simulink model "tesv"  (R2012b)
settings: Solver=ode45  SolverMode=SingleTasking  StartTime=0.0  StopTime=10.0  RelTol=1e-3
libraries: xbsIndex_r4 x837
(part 1 of 6)
settings Model: Creator=tmadden  LastModifiedBy=tmadden
settings DataIOCC: SignalLoggingSaveFormat=ModelDataLogs
settings OptimizationCC: BlockReduction=off  BooleanDataType=off
settings DebuggingCC: SaveWithParameterizedLinksMsg=none  SignalResolutionControl=TryResolveAllWithWarning  SolverPrmCheckMsg=none  MultiTaskDSMMsg=warning  MultiTaskCondExecSysMsg=none  StrictBusMsg=None
settings HardwareCC: TargetUnknown=on
settings RTWCC: IncludeERTFirstTime=on

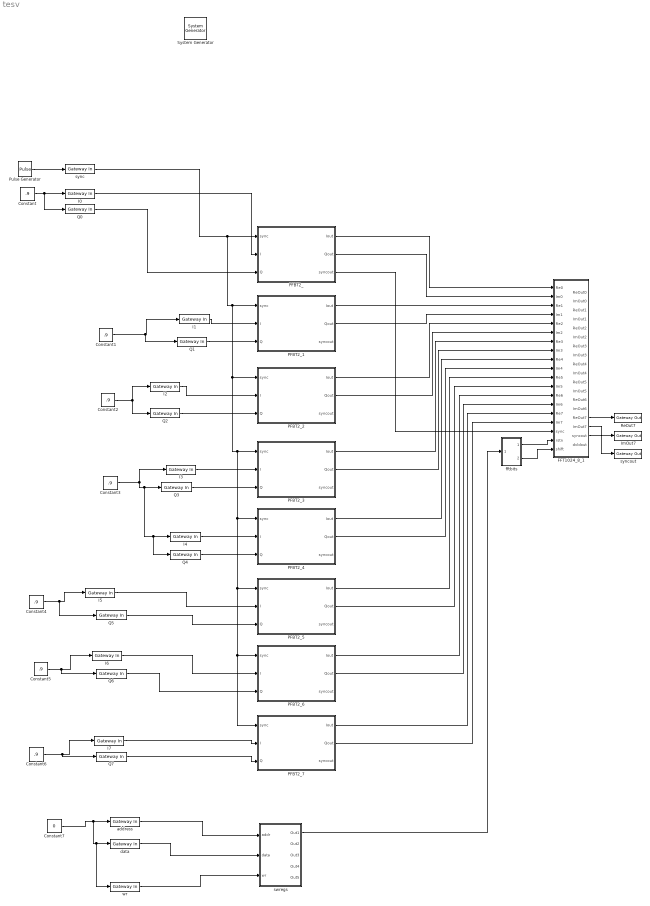
== system tesv ==
  " System Generator" : xbsIndex_r4/ System Generator  Tag=genX  xilinxfamily=zynq  part=xc7z100  speed=-2  package=ffv900  synthesis_tool=XST  clock_wrapper=Clock Enables  directory=./untitled/sysgen  proj_type=Project Navigator  Synth_file=XST Defaults  Impl_file=ISE Defaults  testbench=off  simulink_period=1  sysclk_period=10  dcm_input_clock_period=10  incr_netlist=off  trim_vbits=Everywhere in SubSystem  dbl_ovrd=According to Block Masks  core_generation=According to Block Masks  run_coregen=off  deprecated_control=off  eval_field=0  block_type=sysgen
  Constant{,1..6} (7 alike) : Constant  Value=.9
  Constant7 : Constant  Value=0
  FFT1024_8_1 : Subsystem
  I{0..7} (8 alike) : xbsIndex_r4/Gateway In  gui_display_data_type=Fixed-point  arith_type="Signed  (2's comp)"  n_bits=18  bin_pt=16  preci_type=Single  exp_width=8  frac_width=24  rows=1  columns=1  quantization="Round  (unbiased: +/- Inf)"  overflow=Saturate  period=1  UseAsADC=off  ADCChannel='1'  interface=None  automatic_assignment=on  address_offset=hex2dec('00')  intf_name=''  intf_description=''  timing_constraint=None  locs_specified=off  LOCs={}  io_standard={}  inherit_from_input=off  hdl_port=on  dbl_ovrd=off  block_type=gatewayin
  ImOut7 : xbsIndex_r4/Gateway Out  inherit_from_input=off  hdl_port=on  rows=1  columns=1  UseAsDAC=off  DACChannel='1'  interface=None  automatic_assignment=on  address_offset=hex2dec('00')  intf_name=''  intf_description=''  timing_constraint=None  locs_specified=off  LOCs={}  io_standard={}  block_type=gatewayout
  PFBT2_ : Subsystem
  PFBT2_1 : Subsystem
  PFBT2_2 : Subsystem
  PFBT2_3 : Subsystem
  PFBT2_4 : Subsystem
  PFBT2_5 : Subsystem
  PFBT2_6 : Subsystem
  PFBT2_7 : Subsystem
  Pulse Generator : DiscretePulseGenerator  Period=1024
  Q{0..7} (8 alike) : xbsIndex_r4/Gateway In  gui_display_data_type=Fixed-point  arith_type="Signed  (2's comp)"  n_bits=18  bin_pt=16  preci_type=Single  exp_width=8  frac_width=24  rows=1  columns=1  quantization="Round  (unbiased: +/- Inf)"  overflow=Saturate  period=1  UseAsADC=off  ADCChannel='1'  interface=None  automatic_assignment=on  address_offset=hex2dec('00')  intf_name=''  intf_description=''  timing_constraint=None  locs_specified=off  LOCs={}  io_standard={}  inherit_from_input=off  hdl_port=on  dbl_ovrd=off  block_type=gatewayin
  ReOut7 : xbsIndex_r4/Gateway Out  inherit_from_input=off  hdl_port=on  rows=1  columns=1  UseAsDAC=off  DACChannel='1'  interface=None  automatic_assignment=on  address_offset=hex2dec('00')  intf_name=''  intf_description=''  timing_constraint=None  locs_specified=off  LOCs={}  io_standard={}  block_type=gatewayout
  address : xbsIndex_r4/Gateway In  gui_display_data_type=Fixed-point  arith_type=Unsigned  n_bits=8  bin_pt=0  preci_type=Single  exp_width=8  frac_width=24  rows=1  columns=1  quantization="Round  (unbiased: +/- Inf)"  overflow=Saturate  period=1  UseAsADC=off  ADCChannel='1'  interface=None  automatic_assignment=on  address_offset=hex2dec('00')  intf_name=''  intf_description=''  timing_constraint=None  locs_specified=off  LOCs={}  io_standard={}  inherit_from_input=off  hdl_port=on  dbl_ovrd=off  block_type=gatewayin
  data : xbsIndex_r4/Gateway In  gui_display_data_type=Fixed-point  arith_type=Unsigned  n_bits=32  bin_pt=0  preci_type=Single  exp_width=8  frac_width=24  rows=1  columns=1  quantization="Round  (unbiased: +/- Inf)"  overflow=Saturate  period=1  UseAsADC=off  ADCChannel='1'  interface=None  automatic_assignment=on  address_offset=hex2dec('00')  intf_name=''  intf_description=''  timing_constraint=None  locs_specified=off  LOCs={}  io_standard={}  inherit_from_input=off  hdl_port=on  dbl_ovrd=off  block_type=gatewayin
  fftbits : Subsystem
  swregs : Subsystem
  sync : xbsIndex_r4/Gateway In  gui_display_data_type=Boolean  arith_type=Boolean  n_bits=16  bin_pt=14  preci_type=Single  exp_width=8  frac_width=24  rows=1  columns=1  quantization="Round  (unbiased: +/- Inf)"  overflow=Saturate  period=1  UseAsADC=off  ADCChannel='1'  interface=None  automatic_assignment=on  address_offset=hex2dec('00')  intf_name=''  intf_description=''  timing_constraint=None  locs_specified=off  LOCs={}  io_standard={}  inherit_from_input=off  hdl_port=on  dbl_ovrd=off  block_type=gatewayin
  syncout : xbsIndex_r4/Gateway Out  inherit_from_input=off  hdl_port=on  rows=1  columns=1  UseAsDAC=off  DACChannel='1'  interface=None  automatic_assignment=on  address_offset=hex2dec('00')  intf_name=''  intf_description=''  timing_constraint=None  locs_specified=off  LOCs={}  io_standard={}  block_type=gatewayout
  wr : xbsIndex_r4/Gateway In  gui_display_data_type=Boolean  arith_type=Boolean  n_bits=18  bin_pt=16  preci_type=Single  exp_width=8  frac_width=24  rows=1  columns=1  quantization="Round  (unbiased: +/- Inf)"  overflow=Saturate  period=1  UseAsADC=off  ADCChannel='1'  interface=None  automatic_assignment=on  address_offset=hex2dec('00')  intf_name=''  intf_description=''  timing_constraint=None  locs_specified=off  LOCs={}  io_standard={}  inherit_from_input=off  hdl_port=on  dbl_ovrd=off  block_type=gatewayin
  wires:
  Pulse Generator/1 -> sync/1
  Constant/1 -> Q0/1, I0/1
  sync/1 -> PFBT2_7/1(sync), PFBT2_6/1(sync), PFBT2_5/1(sync), PFBT2_4/1(sync), PFBT2_3/1(sync), PFBT2_2/1(sync), PFBT2_1/1(sync), PFBT2_/1(sync)
  I0/1 -> PFBT2_/2(I)
  Q0/1 -> PFBT2_/3(Q)
  I1/1 -> PFBT2_1/2(I)
  Q1/1 -> PFBT2_1/3(Q)
  I2/1 -> PFBT2_2/2(I)
  Q2/1 -> PFBT2_2/3(Q)
  I3/1 -> PFBT2_3/2(I)
  Q3/1 -> PFBT2_3/3(Q)
  I4/1 -> PFBT2_4/2(I)
  Q4/1 -> PFBT2_4/3(Q)
  I5/1 -> PFBT2_5/2(I)
  Q5/1 -> PFBT2_5/3(Q)
  I6/1 -> PFBT2_6/2(I)
  Q6/1 -> PFBT2_6/3(Q)
  I7/1 -> PFBT2_7/2(I)
  Q7/1 -> PFBT2_7/3(Q)
  Constant6/1 -> Q7/1, I7/1
  Constant5/1 -> Q6/1, I6/1
  Constant4/1 -> Q5/1, I5/1
  Constant3/1 -> Q4/1, I4/1, Q3/1, I3/1
  Constant1/1 -> Q1/1, I1/1
  Constant2/1 -> Q2/1, I2/1
  address/1 -> swregs/1(addr)
  data/1 -> swregs/2(data)
  wr/1 -> swregs/3(wr)
  PFBT2_/1(Iout) -> FFT1024_8_1/1(Re0)
  PFBT2_/2(Qout) -> FFT1024_8_1/2(Im0)
  PFBT2_1/1(Iout) -> FFT1024_8_1/3(Re1)
  PFBT2_1/2(Qout) -> FFT1024_8_1/4(Im1)
  PFBT2_2/1(Iout) -> FFT1024_8_1/5(Re2)
  PFBT2_2/2(Qout) -> FFT1024_8_1/6(Im2)
  PFBT2_3/1(Iout) -> FFT1024_8_1/7(Re3)
  PFBT2_3/2(Qout) -> FFT1024_8_1/8(Im3)
  PFBT2_4/1(Iout) -> FFT1024_8_1/9(Re4)
  PFBT2_4/2(Qout) -> FFT1024_8_1/10(Im4)
  PFBT2_5/1(Iout) -> FFT1024_8_1/11(Re5)
  PFBT2_5/2(Qout) -> FFT1024_8_1/12(Im5)
  PFBT2_6/1(Iout) -> FFT1024_8_1/13(Re6)
  PFBT2_6/2(Qout) -> FFT1024_8_1/14(Im6)
  PFBT2_7/1(Iout) -> FFT1024_8_1/15(Re7)
  PFBT2_7/2(Qout) -> FFT1024_8_1/16(Im7)
  PFBT2_/3(syncout) -> FFT1024_8_1/17(sync)
  fftbits/1(Out1) -> FFT1024_8_1/18(rstn)
  fftbits/2(Out2) -> FFT1024_8_1/19(shift)
  swregs/1(Out1) -> fftbits/1(In1)
  Constant7/1 -> wr/1, data/1, address/1
  FFT1024_8_1/15(ReOut7) -> ReOut7/1
  FFT1024_8_1/16(ImOut7) -> ImOut7/1
  FFT1024_8_1/17(syncout) -> syncout/1

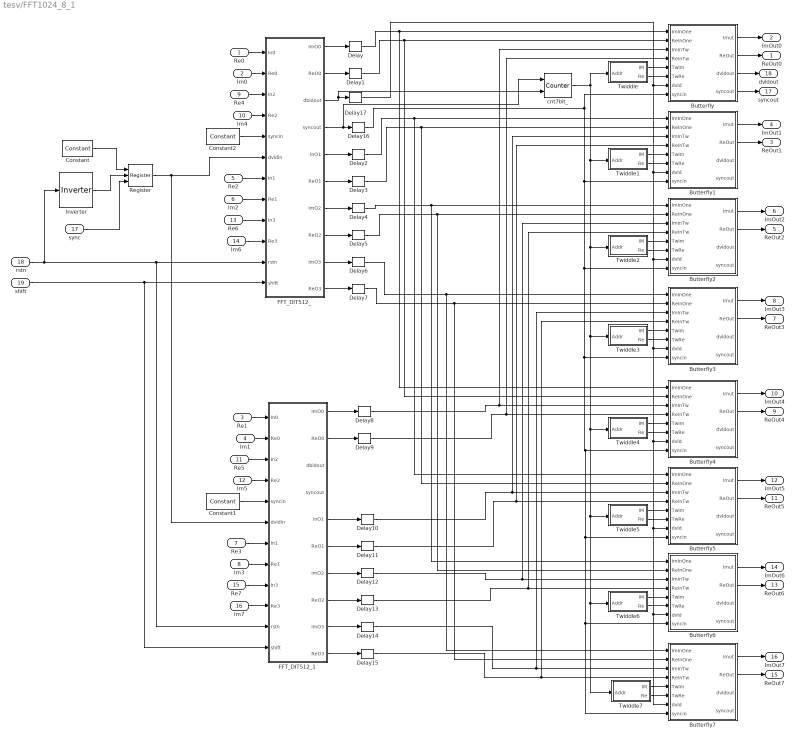
== system tesv/FFT1024_8_1 ==
  Re0 : Inport
  Im0 : Inport  Port=2
  Re1 : Inport  Port=3
  Im1 : Inport  Port=4
  Re2 : Inport  Port=5
  Im2 : Inport  Port=6
  Re3 : Inport  Port=7
  Im3 : Inport  Port=8
  Re4 : Inport  Port=9
  Im4 : Inport  Port=10
  Re5 : Inport  Port=11
  Im5 : Inport  Port=12
  Re6 : Inport  Port=13
  Im6 : Inport  Port=14
  Re7 : Inport  Port=15
  Im7 : Inport  Port=16
  sync : Inport  Port=17
  rstn : Inport  Port=18
  shift : Inport  Port=19
  Butterfly : Subsystem
  Butterfly1 : Subsystem
  Butterfly2 : Subsystem
  Butterfly3 : Subsystem
  Butterfly4 : Subsystem
  Butterfly5 : Subsystem
  Butterfly6 : Subsystem
  Butterfly7 : Subsystem
  Constant : xbsIndex_r4/Constant  const=1  gui_display_data_type=Boolean  arith_type=Boolean  n_bits=16  bin_pt=14  preci_type=Single  exp_width=8  frac_width=24  explicit_period=on  period=1  equ=P=C  opselect=C  inp2=PCIN>>17  opr=+  inp1=P  carry=CIN  dbl_ovrd=off  block_type=constant
  Constant1 : xbsIndex_r4/Constant  const=0  gui_display_data_type=Boolean  arith_type=Boolean  n_bits=16  bin_pt=14  preci_type=Single  exp_width=8  frac_width=24  explicit_period=on  period=1  equ=P=C  opselect=C  inp2=PCIN>>17  opr=+  inp1=P  carry=CIN  dbl_ovrd=off  block_type=constant
  Constant2 : xbsIndex_r4/Constant  const=0  gui_display_data_type=Boolean  arith_type=Boolean  n_bits=16  bin_pt=14  preci_type=Single  exp_width=8  frac_width=24  explicit_period=on  period=1  equ=P=C  opselect=C  inp2=PCIN>>17  opr=+  inp1=P  carry=CIN  dbl_ovrd=off  block_type=constant
  Delay{,1..17} (18 alike) : xbsIndex_r4/Delay  rst=off  infoeditControl=Selection of Reset will increase slice count due to use of real FFs and instead of SRLs  en=off  latency=1  reg_retiming=off  dbl_ovrd=off  block_type=delay
  FFT_DIT512_ : Subsystem
  FFT_DIT512_1 : Subsystem
  Inverter : xbsIndex_r4/Inverter  en=off  latency=0  dbl_ovrd=off  block_type=inv
  Register : xbsIndex_r4/Register  init=0  rst=on  en=on  dbl_ovrd=off  block_type=register
  Twiddle : Subsystem  mask{TFL=1024, NS=8, WS=0}
      mask prompts: TFL "TotFFTLen"; NS "NStreams (1...N)"; WS "WhichStream (0..N-1)"
  Twiddle1 : Subsystem  mask{TFL=1024, NS=8, WS=1}
      mask prompts: TFL "TotFFTLen"; NS "NStreams (1...N)"; WS "WhichStream (0..N-1)"
  Twiddle2 : Subsystem  mask{TFL=1024, NS=8, WS=2}
      mask prompts: TFL "TotFFTLen"; NS "NStreams (1...N)"; WS "WhichStream (0..N-1)"
  Twiddle3 : Subsystem  mask{TFL=1024, NS=8, WS=3}
      mask prompts: TFL "TotFFTLen"; NS "NStreams (1...N)"; WS "WhichStream (0..N-1)"
  Twiddle4 : Subsystem  mask{TFL=1024, NS=8, WS=4}
      mask prompts: TFL "TotFFTLen"; NS "NStreams (1...N)"; WS "WhichStream (0..N-1)"
  Twiddle5 : Subsystem  mask{TFL=1024, NS=8, WS=5}
      mask prompts: TFL "TotFFTLen"; NS "NStreams (1...N)"; WS "WhichStream (0..N-1)"
  Twiddle6 : Subsystem  mask{TFL=1024, NS=8, WS=6}
      mask prompts: TFL "TotFFTLen"; NS "NStreams (1...N)"; WS "WhichStream (0..N-1)"
  Twiddle7 : Subsystem  mask{TFL=1024, NS=8, WS=7}
      mask prompts: TFL "TotFFTLen"; NS "NStreams (1...N)"; WS "WhichStream (0..N-1)"
  cnt7bit_ : xbsIndex_r4/Counter  cnt_type=Free Running  cnt_to=Inf  operation=Up  start_count=0  cnt_by_val=1  arith_type=Unsigned  n_bits=log2(1024/8)  bin_pt=0  load_pin=off  rst=on  en=on  explicit_period=on  period=1  use_behavioral_HDL=off  implementation=Fabric  dbl_ovrd=off  block_type=counter
  ReOut0 : Outport
  ImOut0 : Outport  Port=2
  ReOut1 : Outport  Port=3
  ImOut1 : Outport  Port=4
  ReOut2 : Outport  Port=5
  ImOut2 : Outport  Port=6
  ReOut3 : Outport  Port=7
  ImOut3 : Outport  Port=8
  ReOut4 : Outport  Port=9
  ImOut4 : Outport  Port=10
  ReOut5 : Outport  Port=11
  ImOut5 : Outport  Port=12
  ReOut6 : Outport  Port=13
  ImOut6 : Outport  Port=14
  ReOut7 : Outport  Port=15
  ImOut7 : Outport  Port=16
  syncout : Outport  Port=17
  dvldout : Outport  Port=18
  wires:
  FFT_DIT512_/1(ImO0) -> Delay/1
  FFT_DIT512_/2(ReO0) -> Delay1/1
  Delay/1 -> Butterfly4/1(ImInOne), Butterfly/1(ImInOne)
  Delay1/1 -> Butterfly4/2(ReInOne), Butterfly/2(ReInOne)
  FFT_DIT512_/5(InO1) -> Delay2/1
  Delay2/1 -> Butterfly5/1(ImInOne), Butterfly1/1(ImInOne)
  Delay3/1 -> Butterfly5/2(ReInOne), Butterfly1/2(ReInOne)
  FFT_DIT512_/6(ReO1) -> Delay3/1
  Delay4/1 -> Butterfly6/1(ImInOne), Butterfly2/1(ImInOne)
  Delay5/1 -> Butterfly6/2(ReInOne), Butterfly2/2(ReInOne)
  FFT_DIT512_/7(ImO2) -> Delay4/1
  FFT_DIT512_/8(ReO2) -> Delay5/1
  FFT_DIT512_/9(ImO3) -> Delay6/1
  FFT_DIT512_/10(ReO3) -> Delay7/1
  Delay6/1 -> Butterfly7/1(ImInOne), Butterfly3/1(ImInOne)
  Delay7/1 -> Butterfly7/2(ReInOne), Butterfly3/2(ReInOne)
  FFT_DIT512_1/1(ImO0) -> Delay8/1
  FFT_DIT512_1/2(ReO0) -> Delay9/1
  FFT_DIT512_1/5(InO1) -> Delay10/1
  FFT_DIT512_1/6(ReO1) -> Delay11/1
  FFT_DIT512_1/7(ImO2) -> Delay12/1
  FFT_DIT512_1/8(ReO2) -> Delay13/1
  FFT_DIT512_1/9(ImO3) -> Delay14/1
  FFT_DIT512_1/10(ReO3) -> Delay15/1
  Delay8/1 -> Butterfly/3(ImInTw), Butterfly4/3(ImInTw)
  Delay9/1 -> Butterfly/4(ReInTw), Butterfly4/4(ReInTw)
  Delay10/1 -> Butterfly1/3(ImInTw), Butterfly5/3(ImInTw)
  Delay11/1 -> Butterfly1/4(ReInTw), Butterfly5/4(ReInTw)
  Delay12/1 -> Butterfly2/3(ImInTw), Butterfly6/3(ImInTw)
  Delay13/1 -> Butterfly2/4(ReInTw), Butterfly6/4(ReInTw)
  Delay14/1 -> Butterfly3/3(ImInTw), Butterfly7/3(ImInTw)
  Delay15/1 -> Butterfly3/4(ReInTw), Butterfly7/4(ReInTw)
  Twiddle7/1(IM) -> Butterfly7/5(TwIm)
  Twiddle7/2(Re) -> Butterfly7/6(TwRe)
  Twiddle6/1(IM) -> Butterfly6/5(TwIm)
  Twiddle6/2(Re) -> Butterfly6/6(TwRe)
  Twiddle5/1(IM) -> Butterfly5/5(TwIm)
  Twiddle5/2(Re) -> Butterfly5/6(TwRe)
  Twiddle4/1(IM) -> Butterfly4/5(TwIm)
  Twiddle4/2(Re) -> Butterfly4/6(TwRe)
  Twiddle/1(IM) -> Butterfly/5(TwIm)
  Twiddle/2(Re) -> Butterfly/6(TwRe)
  Twiddle1/1(IM) -> Butterfly1/5(TwIm)
  Twiddle1/2(Re) -> Butterfly1/6(TwRe)
  Twiddle2/1(IM) -> Butterfly2/5(TwIm)
  Twiddle2/2(Re) -> Butterfly2/6(TwRe)
  Twiddle3/1(IM) -> Butterfly3/5(TwIm)
  Twiddle3/2(Re) -> Butterfly3/6(TwRe)
  cnt7bit_/1 -> Twiddle/1(Addr), Twiddle7/1(Addr), Twiddle6/1(Addr), Twiddle5/1(Addr), Twiddle4/1(Addr), Twiddle3/1(Addr), Twiddle2/1(Addr), Twiddle1/1(Addr)
  Inverter/1 -> Register/2
  Constant/1 -> Register/1
  Constant2/1 -> FFT_DIT512_/5(syncin)
  Constant1/1 -> FFT_DIT512_1/5(syncin)
  Register/1 -> FFT_DIT512_1/6(dvldin), FFT_DIT512_/6(dvldin)
  FFT_DIT512_/4(syncout) -> cnt7bit_/1, Delay16/1
  Delay16/1 -> Butterfly7/8(syncin), Butterfly6/8(syncin), Butterfly5/8(syncin), Butterfly4/8(syncin), Butterfly3/8(syncin), Butterfly2/8(syncin), Butterfly1/8(syncin), Butterfly/8(syncin)
  FFT_DIT512_/3(dbldout) -> Delay17/1, cnt7bit_/2
  Delay17/1 -> Butterfly7/7(dvld), Butterfly6/7(dvld), Butterfly5/7(dvld), Butterfly4/7(dvld), Butterfly3/7(dvld), Butterfly2/7(dvld), Butterfly1/7(dvld), Butterfly/7(dvld)
  Im7/1 -> FFT_DIT512_1/10(Re3)
  Re7/1 -> FFT_DIT512_1/9(In3)
  Re3/1 -> FFT_DIT512_1/7(In1)
  Im3/1 -> FFT_DIT512_1/8(Re1)
  Im5/1 -> FFT_DIT512_1/4(Re2)
  Re5/1 -> FFT_DIT512_1/3(In2)
  Im1/1 -> FFT_DIT512_1/2(Re0)
  Re1/1 -> FFT_DIT512_1/1(In0)
  Im6/1 -> FFT_DIT512_/10(Re3)
  Re6/1 -> FFT_DIT512_/9(In3)
  Im2/1 -> FFT_DIT512_/8(Re1)
  Re2/1 -> FFT_DIT512_/7(In1)
  Re0/1 -> FFT_DIT512_/1(In0)
  Im0/1 -> FFT_DIT512_/2(Re0)
  Re4/1 -> FFT_DIT512_/3(In2)
  Im4/1 -> FFT_DIT512_/4(Re2)
  sync/1 -> Register/3
  rstn/1 -> Inverter/1, FFT_DIT512_1/11(rstn), FFT_DIT512_/11(rstn)
  shift/1 -> FFT_DIT512_1/12(shift), FFT_DIT512_/12(shift)
  Butterfly/2(ReOut) -> ReOut0/1
  Butterfly/1(Imut) -> ImOut0/1
  Butterfly1/1(Imut) -> ImOut1/1
  Butterfly1/2(ReOut) -> ReOut1/1
  Butterfly2/1(Imut) -> ImOut2/1
  Butterfly2/2(ReOut) -> ReOut2/1
  Butterfly3/1(Imut) -> ImOut3/1
  Butterfly3/2(ReOut) -> ReOut3/1
  Butterfly4/1(Imut) -> ImOut4/1
  Butterfly4/2(ReOut) -> ReOut4/1
  Butterfly5/1(Imut) -> ImOut5/1
  Butterfly5/2(ReOut) -> ReOut5/1
  Butterfly6/1(Imut) -> ImOut6/1
  Butterfly6/2(ReOut) -> ReOut6/1
  Butterfly7/1(Imut) -> ImOut7/1
  Butterfly7/2(ReOut) -> ReOut7/1
  Butterfly/3(dvldout) -> dvldout/1
  Butterfly/4(syncout) -> syncout/1

== system tesv/PFBT2_ ==
  sync : Inport
  I : Inport  Port=2
  Q : Inport  Port=3
  AddSub : xbsIndex_r4/AddSub  mode=Addition  use_carryin=off  use_carryout=off  en=off  latency=1  precision=Full  arith_type=Unsigned  n_bits=16  bin_pt=14  quantization=Truncate  overflow=Wrap  use_behavioral_HDL=off  hw_selection=Fabric  pipelined=off  dbl_ovrd=off  block_type=addsub
  AddSub1 : xbsIndex_r4/AddSub  mode=Addition  use_carryin=off  use_carryout=off  en=off  latency=1  precision=Full  arith_type=Unsigned  n_bits=16  bin_pt=14  quantization=Truncate  overflow=Wrap  use_behavioral_HDL=off  hw_selection=Fabric  pipelined=off  dbl_ovrd=off  block_type=addsub
  CoefAddr_ : Subsystem  mask{FL=1024, NS=8}
      mask prompts: FL "FilterLen (FFT Len)"; NS "NumStreams"
  Delay_ : Subsystem  mask{FL=1024, NS=8}
      mask prompts: FL "FiltLen (FFT Len)"; NS "NumStreams"
  Delay_1 : Subsystem  mask{FL=1024, NS=8}
      mask prompts: FL "FiltLen (FFT Len)"; NS "NumStreams"
  TapIQ_1 : Subsystem  mask{FL=1024, WS=0, NS=8, WT=1, NT=2}
      mask prompts: FL "FilterLen"; WS "WhichStream(0..3)"; NS "NStreams"; WT "WhichTap (0..3)"; NT "NumTaps"
  TapIQ_2 : Subsystem  mask{FL=1024, WS=0, NS=8, WT=0, NT=2}
      mask prompts: FL "FilterLen"; WS "WhichStream(0..3)"; NS "NStreams"; WT "WhichTap (0..3)"; NT "NumTaps"
  Iout : Outport
  Qout : Outport  Port=2
  syncout : Outport  Port=3
  wires:
  TapIQ_1/4(syncout) -> syncout/1
  Delay_/1(Iout) -> TapIQ_1/1(Iin)
  Delay_/2(Qout) -> TapIQ_1/2(Qin)
  TapIQ_2/1(Iout) -> Delay_1/1(Iin)
  TapIQ_1/1(Iout) -> AddSub/2
  Delay_1/1(Iout) -> AddSub/1
  Delay_1/2(Qout) -> AddSub1/1
  TapIQ_1/2(Qout) -> AddSub1/2
  Delay_/3(addrout) -> TapIQ_1/3(coefaddr)
  CoefAddr_/1(Addr) -> Delay_/3(addrin), TapIQ_2/3(coefaddr)
  Q/1 -> CoefAddr_/3(Qin)
  I/1 -> CoefAddr_/2(Iin)
  sync/1 -> CoefAddr_/1(sync)
  CoefAddr_/2(Iout) -> TapIQ_2/1(Iin), Delay_/1(Iin)
  CoefAddr_/3(Qout) -> Delay_/2(Qin), TapIQ_2/2(Qin)
  TapIQ_2/4(syncout) -> Delay_1/4(sync)
  CoefAddr_/4(syncout) -> TapIQ_2/4(sync), Delay_/4(sync)
  Delay_/4(syncout) -> TapIQ_1/4(sync)
  AddSub/1 -> Iout/1
  AddSub1/1 -> Qout/1
  TapIQ_2/2(Qout) -> Delay_1/2(Qin)
  TapIQ_2/3(coefaddrout) -> Delay_1/3(addrin)

== system tesv/PFBT2_1 ==
  sync : Inport
  I : Inport  Port=2
  Q : Inport  Port=3
  AddSub : xbsIndex_r4/AddSub  mode=Addition  use_carryin=off  use_carryout=off  en=off  latency=1  precision=Full  arith_type=Unsigned  n_bits=16  bin_pt=14  quantization=Truncate  overflow=Wrap  use_behavioral_HDL=off  hw_selection=Fabric  pipelined=off  dbl_ovrd=off  block_type=addsub
  AddSub1 : xbsIndex_r4/AddSub  mode=Addition  use_carryin=off  use_carryout=off  en=off  latency=1  precision=Full  arith_type=Unsigned  n_bits=16  bin_pt=14  quantization=Truncate  overflow=Wrap  use_behavioral_HDL=off  hw_selection=Fabric  pipelined=off  dbl_ovrd=off  block_type=addsub
  CoefAddr_ : Subsystem  mask{FL=1024, NS=8}
      mask prompts: FL "FilterLen (FFT Len)"; NS "NumStreams"
  Delay_ : Subsystem  mask{FL=1024, NS=8}
      mask prompts: FL "FiltLen (FFT Len)"; NS "NumStreams"
  Delay_1 : Subsystem  mask{FL=1024, NS=8}
      mask prompts: FL "FiltLen (FFT Len)"; NS "NumStreams"
  TapIQ_1 : Subsystem  mask{FL=1024, WS=1, NS=8, WT=1, NT=2}
      mask prompts: FL "FilterLen"; WS "WhichStream(0..3)"; NS "NStreams"; WT "WhichTap (0..3)"; NT "NumTaps"
  TapIQ_2 : Subsystem  mask{FL=1024, WS=1, NS=8, WT=0, NT=2}
      mask prompts: FL "FilterLen"; WS "WhichStream(0..3)"; NS "NStreams"; WT "WhichTap (0..3)"; NT "NumTaps"
  Iout : Outport
  Qout : Outport  Port=2
  syncout : Outport  Port=3
  wires:
  TapIQ_1/4(syncout) -> syncout/1
  Delay_/1(Iout) -> TapIQ_1/1(Iin)
  Delay_/2(Qout) -> TapIQ_1/2(Qin)
  TapIQ_2/1(Iout) -> Delay_1/1(Iin)
  TapIQ_1/1(Iout) -> AddSub/2
  Delay_1/1(Iout) -> AddSub/1
  Delay_1/2(Qout) -> AddSub1/1
  TapIQ_1/2(Qout) -> AddSub1/2
  Delay_/3(addrout) -> TapIQ_1/3(coefaddr)
  CoefAddr_/1(Addr) -> Delay_/3(addrin), TapIQ_2/3(coefaddr)
  Q/1 -> CoefAddr_/3(Qin)
  I/1 -> CoefAddr_/2(Iin)
  sync/1 -> CoefAddr_/1(sync)
  CoefAddr_/2(Iout) -> TapIQ_2/1(Iin), Delay_/1(Iin)
  CoefAddr_/3(Qout) -> Delay_/2(Qin), TapIQ_2/2(Qin)
  TapIQ_2/4(syncout) -> Delay_1/4(sync)
  CoefAddr_/4(syncout) -> TapIQ_2/4(sync), Delay_/4(sync)
  Delay_/4(syncout) -> TapIQ_1/4(sync)
  AddSub/1 -> Iout/1
  AddSub1/1 -> Qout/1
  TapIQ_2/2(Qout) -> Delay_1/2(Qin)
  TapIQ_2/3(coefaddrout) -> Delay_1/3(addrin)

== system tesv/PFBT2_2 ==
  sync : Inport
  I : Inport  Port=2
  Q : Inport  Port=3
  AddSub : xbsIndex_r4/AddSub  mode=Addition  use_carryin=off  use_carryout=off  en=off  latency=1  precision=Full  arith_type=Unsigned  n_bits=16  bin_pt=14  quantization=Truncate  overflow=Wrap  use_behavioral_HDL=off  hw_selection=Fabric  pipelined=off  dbl_ovrd=off  block_type=addsub
  AddSub1 : xbsIndex_r4/AddSub  mode=Addition  use_carryin=off  use_carryout=off  en=off  latency=1  precision=Full  arith_type=Unsigned  n_bits=16  bin_pt=14  quantization=Truncate  overflow=Wrap  use_behavioral_HDL=off  hw_selection=Fabric  pipelined=off  dbl_ovrd=off  block_type=addsub
  CoefAddr_ : Subsystem  mask{FL=1024, NS=8}
      mask prompts: FL "FilterLen (FFT Len)"; NS "NumStreams"
  Delay_ : Subsystem  mask{FL=512, NS=2}
      mask prompts: FL "FiltLen (FFT Len)"; NS "NumStreams"
  Delay_1 : Subsystem  mask{FL=1024, NS=8}
      mask prompts: FL "FiltLen (FFT Len)"; NS "NumStreams"
  TapIQ_1 : Subsystem  mask{FL=1024, WS=2, NS=8, WT=1, NT=2}
      mask prompts: FL "FilterLen"; WS "WhichStream(0..3)"; NS "NStreams"; WT "WhichTap (0..3)"; NT "NumTaps"
  TapIQ_2 : Subsystem  mask{FL=1024, WS=2, NS=8, WT=0, NT=2}
      mask prompts: FL "FilterLen"; WS "WhichStream(0..3)"; NS "NStreams"; WT "WhichTap (0..3)"; NT "NumTaps"
  Iout : Outport
  Qout : Outport  Port=2
  syncout : Outport  Port=3
  wires:
  TapIQ_1/4(syncout) -> syncout/1
  Delay_/1(Iout) -> TapIQ_1/1(Iin)
  Delay_/2(Qout) -> TapIQ_1/2(Qin)
  TapIQ_2/1(Iout) -> Delay_1/1(Iin)
  TapIQ_1/1(Iout) -> AddSub/2
  Delay_1/1(Iout) -> AddSub/1
  Delay_1/2(Qout) -> AddSub1/1
  TapIQ_1/2(Qout) -> AddSub1/2
  Delay_/3(addrout) -> TapIQ_1/3(coefaddr)
  CoefAddr_/1(Addr) -> Delay_/3(addrin), TapIQ_2/3(coefaddr)
  Q/1 -> CoefAddr_/3(Qin)
  I/1 -> CoefAddr_/2(Iin)
  sync/1 -> CoefAddr_/1(sync)
  CoefAddr_/2(Iout) -> TapIQ_2/1(Iin), Delay_/1(Iin)
  CoefAddr_/3(Qout) -> Delay_/2(Qin), TapIQ_2/2(Qin)
  TapIQ_2/4(syncout) -> Delay_1/4(sync)
  CoefAddr_/4(syncout) -> TapIQ_2/4(sync), Delay_/4(sync)
  Delay_/4(syncout) -> TapIQ_1/4(sync)
  AddSub/1 -> Iout/1
  AddSub1/1 -> Qout/1
  TapIQ_2/2(Qout) -> Delay_1/2(Qin)
  TapIQ_2/3(coefaddrout) -> Delay_1/3(addrin)

== system tesv/PFBT2_3 ==
  sync : Inport
  I : Inport  Port=2
  Q : Inport  Port=3
  AddSub : xbsIndex_r4/AddSub  mode=Addition  use_carryin=off  use_carryout=off  en=off  latency=1  precision=Full  arith_type=Unsigned  n_bits=16  bin_pt=14  quantization=Truncate  overflow=Wrap  use_behavioral_HDL=off  hw_selection=Fabric  pipelined=off  dbl_ovrd=off  block_type=addsub
  AddSub1 : xbsIndex_r4/AddSub  mode=Addition  use_carryin=off  use_carryout=off  en=off  latency=1  precision=Full  arith_type=Unsigned  n_bits=16  bin_pt=14  quantization=Truncate  overflow=Wrap  use_behavioral_HDL=off  hw_selection=Fabric  pipelined=off  dbl_ovrd=off  block_type=addsub
  CoefAddr_ : Subsystem  mask{FL=1024, NS=8}
      mask prompts: FL "FilterLen (FFT Len)"; NS "NumStreams"
  Delay_ : Subsystem  mask{FL=1024, NS=8}
      mask prompts: FL "FiltLen (FFT Len)"; NS "NumStreams"
  Delay_1 : Subsystem  mask{FL=1024, NS=8}
      mask prompts: FL "FiltLen (FFT Len)"; NS "NumStreams"
  TapIQ_1 : Subsystem  mask{FL=1024, WS=3, NS=8, WT=1, NT=2}
      mask prompts: FL "FilterLen"; WS "WhichStream(0..3)"; NS "NStreams"; WT "WhichTap (0..3)"; NT "NumTaps"
  TapIQ_2 : Subsystem  mask{FL=1024, WS=3, NS=8, WT=0, NT=2}
      mask prompts: FL "FilterLen"; WS "WhichStream(0..3)"; NS "NStreams"; WT "WhichTap (0..3)"; NT "NumTaps"
  Iout : Outport
  Qout : Outport  Port=2
  syncout : Outport  Port=3
  wires:
  TapIQ_1/4(syncout) -> syncout/1
  Delay_/1(Iout) -> TapIQ_1/1(Iin)
  Delay_/2(Qout) -> TapIQ_1/2(Qin)
  TapIQ_2/1(Iout) -> Delay_1/1(Iin)
  TapIQ_1/1(Iout) -> AddSub/2
  Delay_1/1(Iout) -> AddSub/1
  Delay_1/2(Qout) -> AddSub1/1
  TapIQ_1/2(Qout) -> AddSub1/2
  Delay_/3(addrout) -> TapIQ_1/3(coefaddr)
  CoefAddr_/1(Addr) -> Delay_/3(addrin), TapIQ_2/3(coefaddr)
  Q/1 -> CoefAddr_/3(Qin)
  I/1 -> CoefAddr_/2(Iin)
  sync/1 -> CoefAddr_/1(sync)
  CoefAddr_/2(Iout) -> TapIQ_2/1(Iin), Delay_/1(Iin)
  CoefAddr_/3(Qout) -> Delay_/2(Qin), TapIQ_2/2(Qin)
  TapIQ_2/4(syncout) -> Delay_1/4(sync)
  CoefAddr_/4(syncout) -> TapIQ_2/4(sync), Delay_/4(sync)
  Delay_/4(syncout) -> TapIQ_1/4(sync)
  AddSub/1 -> Iout/1
  AddSub1/1 -> Qout/1
  TapIQ_2/2(Qout) -> Delay_1/2(Qin)
  TapIQ_2/3(coefaddrout) -> Delay_1/3(addrin)

== system tesv/PFBT2_4 ==
  sync : Inport
  I : Inport  Port=2
  Q : Inport  Port=3
  AddSub : xbsIndex_r4/AddSub  mode=Addition  use_carryin=off  use_carryout=off  en=off  latency=1  precision=Full  arith_type=Unsigned  n_bits=16  bin_pt=14  quantization=Truncate  overflow=Wrap  use_behavioral_HDL=off  hw_selection=Fabric  pipelined=off  dbl_ovrd=off  block_type=addsub
  AddSub1 : xbsIndex_r4/AddSub  mode=Addition  use_carryin=off  use_carryout=off  en=off  latency=1  precision=Full  arith_type=Unsigned  n_bits=16  bin_pt=14  quantization=Truncate  overflow=Wrap  use_behavioral_HDL=off  hw_selection=Fabric  pipelined=off  dbl_ovrd=off  block_type=addsub
  CoefAddr_ : Subsystem  mask{FL=1024, NS=8}
      mask prompts: FL "FilterLen (FFT Len)"; NS "NumStreams"
  Delay_ : Subsystem  mask{FL=1024, NS=8}
      mask prompts: FL "FiltLen (FFT Len)"; NS "NumStreams"
  Delay_1 : Subsystem  mask{FL=1024, NS=8}
      mask prompts: FL "FiltLen (FFT Len)"; NS "NumStreams"
  TapIQ_1 : Subsystem  mask{FL=1024, WS=4, NS=8, WT=1, NT=2}
      mask prompts: FL "FilterLen"; WS "WhichStream(0..3)"; NS "NStreams"; WT "WhichTap (0..3)"; NT "NumTaps"
  TapIQ_2 : Subsystem  mask{FL=1024, WS=4, NS=8, WT=0, NT=2}
      mask prompts: FL "FilterLen"; WS "WhichStream(0..3)"; NS "NStreams"; WT "WhichTap (0..3)"; NT "NumTaps"
  Iout : Outport
  Qout : Outport  Port=2
  syncout : Outport  Port=3
  wires:
  TapIQ_1/4(syncout) -> syncout/1
  Delay_/1(Iout) -> TapIQ_1/1(Iin)
  Delay_/2(Qout) -> TapIQ_1/2(Qin)
  TapIQ_2/1(Iout) -> Delay_1/1(Iin)
  TapIQ_1/1(Iout) -> AddSub/2
  Delay_1/1(Iout) -> AddSub/1
  Delay_1/2(Qout) -> AddSub1/1
  TapIQ_1/2(Qout) -> AddSub1/2
  Delay_/3(addrout) -> TapIQ_1/3(coefaddr)
  CoefAddr_/1(Addr) -> Delay_/3(addrin), TapIQ_2/3(coefaddr)
  Q/1 -> CoefAddr_/3(Qin)
  I/1 -> CoefAddr_/2(Iin)
  sync/1 -> CoefAddr_/1(sync)
  CoefAddr_/2(Iout) -> TapIQ_2/1(Iin), Delay_/1(Iin)
  CoefAddr_/3(Qout) -> Delay_/2(Qin), TapIQ_2/2(Qin)
  TapIQ_2/4(syncout) -> Delay_1/4(sync)
  CoefAddr_/4(syncout) -> TapIQ_2/4(sync), Delay_/4(sync)
  Delay_/4(syncout) -> TapIQ_1/4(sync)
  AddSub/1 -> Iout/1
  AddSub1/1 -> Qout/1
  TapIQ_2/2(Qout) -> Delay_1/2(Qin)
  TapIQ_2/3(coefaddrout) -> Delay_1/3(addrin)

== system tesv/PFBT2_5 ==
  sync : Inport
  I : Inport  Port=2
  Q : Inport  Port=3
  AddSub : xbsIndex_r4/AddSub  mode=Addition  use_carryin=off  use_carryout=off  en=off  latency=1  precision=Full  arith_type=Unsigned  n_bits=16  bin_pt=14  quantization=Truncate  overflow=Wrap  use_behavioral_HDL=off  hw_selection=Fabric  pipelined=off  dbl_ovrd=off  block_type=addsub
  AddSub1 : xbsIndex_r4/AddSub  mode=Addition  use_carryin=off  use_carryout=off  en=off  latency=1  precision=Full  arith_type=Unsigned  n_bits=16  bin_pt=14  quantization=Truncate  overflow=Wrap  use_behavioral_HDL=off  hw_selection=Fabric  pipelined=off  dbl_ovrd=off  block_type=addsub
  CoefAddr_ : Subsystem  mask{FL=1024, NS=8}
      mask prompts: FL "FilterLen (FFT Len)"; NS "NumStreams"
  Delay_ : Subsystem  mask{FL=1024, NS=8}
      mask prompts: FL "FiltLen (FFT Len)"; NS "NumStreams"
  Delay_1 : Subsystem  mask{FL=1024, NS=8}
      mask prompts: FL "FiltLen (FFT Len)"; NS "NumStreams"
  TapIQ_1 : Subsystem  mask{FL=1024, WS=5, NS=8, WT=1, NT=2}
      mask prompts: FL "FilterLen"; WS "WhichStream(0..3)"; NS "NStreams"; WT "WhichTap (0..3)"; NT "NumTaps"
  TapIQ_2 : Subsystem  mask{FL=1024, WS=5, NS=8, WT=0, NT=2}
      mask prompts: FL "FilterLen"; WS "WhichStream(0..3)"; NS "NStreams"; WT "WhichTap (0..3)"; NT "NumTaps"
  Iout : Outport
  Qout : Outport  Port=2
  syncout : Outport  Port=3
  wires:
  TapIQ_1/4(syncout) -> syncout/1
  Delay_/1(Iout) -> TapIQ_1/1(Iin)
  Delay_/2(Qout) -> TapIQ_1/2(Qin)
  TapIQ_2/1(Iout) -> Delay_1/1(Iin)
  TapIQ_1/1(Iout) -> AddSub/2
  Delay_1/1(Iout) -> AddSub/1
  Delay_1/2(Qout) -> AddSub1/1
  TapIQ_1/2(Qout) -> AddSub1/2
  Delay_/3(addrout) -> TapIQ_1/3(coefaddr)
  CoefAddr_/1(Addr) -> Delay_/3(addrin), TapIQ_2/3(coefaddr)
  Q/1 -> CoefAddr_/3(Qin)
  I/1 -> CoefAddr_/2(Iin)
  sync/1 -> CoefAddr_/1(sync)
  CoefAddr_/2(Iout) -> TapIQ_2/1(Iin), Delay_/1(Iin)
  CoefAddr_/3(Qout) -> Delay_/2(Qin), TapIQ_2/2(Qin)
  TapIQ_2/4(syncout) -> Delay_1/4(sync)
  CoefAddr_/4(syncout) -> TapIQ_2/4(sync), Delay_/4(sync)
  Delay_/4(syncout) -> TapIQ_1/4(sync)
  AddSub/1 -> Iout/1
  AddSub1/1 -> Qout/1
  TapIQ_2/2(Qout) -> Delay_1/2(Qin)
  TapIQ_2/3(coefaddrout) -> Delay_1/3(addrin)

== system tesv/PFBT2_6 ==
  sync : Inport
  I : Inport  Port=2
  Q : Inport  Port=3
  AddSub : xbsIndex_r4/AddSub  mode=Addition  use_carryin=off  use_carryout=off  en=off  latency=1  precision=Full  arith_type=Unsigned  n_bits=16  bin_pt=14  quantization=Truncate  overflow=Wrap  use_behavioral_HDL=off  hw_selection=Fabric  pipelined=off  dbl_ovrd=off  block_type=addsub
  AddSub1 : xbsIndex_r4/AddSub  mode=Addition  use_carryin=off  use_carryout=off  en=off  latency=1  precision=Full  arith_type=Unsigned  n_bits=16  bin_pt=14  quantization=Truncate  overflow=Wrap  use_behavioral_HDL=off  hw_selection=Fabric  pipelined=off  dbl_ovrd=off  block_type=addsub
  CoefAddr_ : Subsystem  mask{FL=1024, NS=8}
      mask prompts: FL "FilterLen (FFT Len)"; NS "NumStreams"
  Delay_ : Subsystem  mask{FL=1024, NS=8}
      mask prompts: FL "FiltLen (FFT Len)"; NS "NumStreams"
  Delay_1 : Subsystem  mask{FL=1024, NS=8}
      mask prompts: FL "FiltLen (FFT Len)"; NS "NumStreams"
  TapIQ_1 : Subsystem  mask{FL=1024, WS=6, NS=8, WT=1, NT=2}
      mask prompts: FL "FilterLen"; WS "WhichStream(0..3)"; NS "NStreams"; WT "WhichTap (0..3)"; NT "NumTaps"
  TapIQ_2 : Subsystem  mask{FL=1024, WS=6, NS=8, WT=0, NT=2}
      mask prompts: FL "FilterLen"; WS "WhichStream(0..3)"; NS "NStreams"; WT "WhichTap (0..3)"; NT "NumTaps"
  Iout : Outport
  Qout : Outport  Port=2
  syncout : Outport  Port=3
  wires:
  TapIQ_1/4(syncout) -> syncout/1
  Delay_/1(Iout) -> TapIQ_1/1(Iin)
  Delay_/2(Qout) -> TapIQ_1/2(Qin)
  TapIQ_2/1(Iout) -> Delay_1/1(Iin)
  TapIQ_1/1(Iout) -> AddSub/2
  Delay_1/1(Iout) -> AddSub/1
  Delay_1/2(Qout) -> AddSub1/1
  TapIQ_1/2(Qout) -> AddSub1/2
  Delay_/3(addrout) -> TapIQ_1/3(coefaddr)
  CoefAddr_/1(Addr) -> Delay_/3(addrin), TapIQ_2/3(coefaddr)
  Q/1 -> CoefAddr_/3(Qin)
  I/1 -> CoefAddr_/2(Iin)
  sync/1 -> CoefAddr_/1(sync)
  CoefAddr_/2(Iout) -> TapIQ_2/1(Iin), Delay_/1(Iin)
  CoefAddr_/3(Qout) -> Delay_/2(Qin), TapIQ_2/2(Qin)
  TapIQ_2/4(syncout) -> Delay_1/4(sync)
  CoefAddr_/4(syncout) -> TapIQ_2/4(sync), Delay_/4(sync)
  Delay_/4(syncout) -> TapIQ_1/4(sync)
  AddSub/1 -> Iout/1
  AddSub1/1 -> Qout/1
  TapIQ_2/2(Qout) -> Delay_1/2(Qin)
  TapIQ_2/3(coefaddrout) -> Delay_1/3(addrin)

== system tesv/PFBT2_7 ==
  sync : Inport
  I : Inport  Port=2
  Q : Inport  Port=3
  AddSub : xbsIndex_r4/AddSub  mode=Addition  use_carryin=off  use_carryout=off  en=off  latency=1  precision=Full  arith_type=Unsigned  n_bits=16  bin_pt=14  quantization=Truncate  overflow=Wrap  use_behavioral_HDL=off  hw_selection=Fabric  pipelined=off  dbl_ovrd=off  block_type=addsub
  AddSub1 : xbsIndex_r4/AddSub  mode=Addition  use_carryin=off  use_carryout=off  en=off  latency=1  precision=Full  arith_type=Unsigned  n_bits=16  bin_pt=14  quantization=Truncate  overflow=Wrap  use_behavioral_HDL=off  hw_selection=Fabric  pipelined=off  dbl_ovrd=off  block_type=addsub
  CoefAddr_ : Subsystem  mask{FL=1024, NS=8}
      mask prompts: FL "FilterLen (FFT Len)"; NS "NumStreams"
  Delay_ : Subsystem  mask{FL=1024, NS=8}
      mask prompts: FL "FiltLen (FFT Len)"; NS "NumStreams"
  Delay_1 : Subsystem  mask{FL=1024, NS=8}
      mask prompts: FL "FiltLen (FFT Len)"; NS "NumStreams"
  TapIQ_1 : Subsystem  mask{FL=1024, WS=7, NS=8, WT=1, NT=2}
      mask prompts: FL "FilterLen"; WS "WhichStream(0..3)"; NS "NStreams"; WT "WhichTap (0..3)"; NT "NumTaps"
  TapIQ_2 : Subsystem  mask{FL=1024, WS=7, NS=8, WT=0, NT=2}
      mask prompts: FL "FilterLen"; WS "WhichStream(0..3)"; NS "NStreams"; WT "WhichTap (0..3)"; NT "NumTaps"
  Iout : Outport
  Qout : Outport  Port=2
  syncout : Outport  Port=3
  wires:
  TapIQ_1/4(syncout) -> syncout/1
  Delay_/1(Iout) -> TapIQ_1/1(Iin)
  Delay_/2(Qout) -> TapIQ_1/2(Qin)
  TapIQ_2/1(Iout) -> Delay_1/1(Iin)
  TapIQ_1/1(Iout) -> AddSub/2
  Delay_1/1(Iout) -> AddSub/1
  Delay_1/2(Qout) -> AddSub1/1
  TapIQ_1/2(Qout) -> AddSub1/2
  Delay_/3(addrout) -> TapIQ_1/3(coefaddr)
  CoefAddr_/1(Addr) -> Delay_/3(addrin), TapIQ_2/3(coefaddr)
  Q/1 -> CoefAddr_/3(Qin)
  I/1 -> CoefAddr_/2(Iin)
  sync/1 -> CoefAddr_/1(sync)
  CoefAddr_/2(Iout) -> TapIQ_2/1(Iin), Delay_/1(Iin)
  CoefAddr_/3(Qout) -> Delay_/2(Qin), TapIQ_2/2(Qin)
  TapIQ_2/4(syncout) -> Delay_1/4(sync)
  CoefAddr_/4(syncout) -> TapIQ_2/4(sync), Delay_/4(sync)
  Delay_/4(syncout) -> TapIQ_1/4(sync)
  AddSub/1 -> Iout/1
  AddSub1/1 -> Qout/1
  TapIQ_2/2(Qout) -> Delay_1/2(Qin)
  TapIQ_2/3(coefaddrout) -> Delay_1/3(addrin)

== system tesv/fftbits ==
  In1 : Inport
  Inverter : xbsIndex_r4/Inverter  en=off  latency=1  dbl_ovrd=off  block_type=inv
  Slice : xbsIndex_r4/Slice  nbits=1  boolean_output=on  mode=Lower Bit Location + Width  bit1=0  base1=MSB of Input  bit0=0  base0=LSB of Input  dbl_ovrd=off  block_type=slice
  Slice1 : xbsIndex_r4/Slice  nbits=4  boolean_output=off  mode=Lower Bit Location + Width  bit1=0  base1=LSB of Input  bit0=1  base0=LSB of Input  dbl_ovrd=off  block_type=slice
  Out1 : Outport
  Out2 : Outport  Port=2
  wires:
  In1/1 -> Slice1/1, Slice/1
  Inverter/1 -> Out1/1
  Slice/1 -> Inverter/1
  Slice1/1 -> Out2/1

== system tesv/swregs ==
  addr : Inport
  data : Inport  Port=2
  wr : Inport  Port=3
  Constant10 : xbsIndex_r4/Constant  const=3  gui_display_data_type=Fixed-point  arith_type=Unsigned  n_bits=8  bin_pt=0  preci_type=Single  exp_width=8  frac_width=24  explicit_period=on  period=1  equ=P=C  opselect=C  inp2=PCIN>>17  opr=+  inp1=P  carry=CIN  dbl_ovrd=off  block_type=constant
  Constant11 : xbsIndex_r4/Constant  const=4  gui_display_data_type=Fixed-point  arith_type=Unsigned  n_bits=8  bin_pt=0  preci_type=Single  exp_width=8  frac_width=24  explicit_period=on  period=1  equ=P=C  opselect=C  inp2=PCIN>>17  opr=+  inp1=P  carry=CIN  dbl_ovrd=off  block_type=constant
  Constant7 : xbsIndex_r4/Constant  const=0  gui_display_data_type=Fixed-point  arith_type=Unsigned  n_bits=8  bin_pt=0  preci_type=Single  exp_width=8  frac_width=24  explicit_period=on  period=1  equ=P=C  opselect=C  inp2=PCIN>>17  opr=+  inp1=P  carry=CIN  dbl_ovrd=off  block_type=constant
  Constant8 : xbsIndex_r4/Constant  const=1  gui_display_data_type=Fixed-point  arith_type=Unsigned  n_bits=8  bin_pt=0  preci_type=Single  exp_width=8  frac_width=24  explicit_period=on  period=1  equ=P=C  opselect=C  inp2=PCIN>>17  opr=+  inp1=P  carry=CIN  dbl_ovrd=off  block_type=constant
  Constant9 : xbsIndex_r4/Constant  const=2  gui_display_data_type=Fixed-point  arith_type=Unsigned  n_bits=8  bin_pt=0  preci_type=Single  exp_width=8  frac_width=24  explicit_period=on  period=1  equ=P=C  opselect=C  inp2=PCIN>>17  opr=+  inp1=P  carry=CIN  dbl_ovrd=off  block_type=constant
  swregin_ : Subsystem
  swregin_1 : Subsystem
  swregin_2 : Subsystem
  swregin_3 : Subsystem
  swregin_4 : Subsystem
  Out1 : Outport
  Out2 : Outport  Port=2
  Out3 : Outport  Port=3
  Out4 : Outport  Port=4
  Out5 : Outport  Port=5
  wires:
  wr/1 -> swregin_/4(wr), swregin_1/4(wr), swregin_2/4(wr), swregin_3/4(wr), swregin_4/4(wr)
  Constant11/1 -> swregin_4/3(myaddress)
  swregin_4/1(dataout) -> Out5/1
  swregin_2/1(dataout) -> Out3/1
  Constant7/1 -> swregin_/3(myaddress)
  Constant10/1 -> swregin_3/3(myaddress)
  data/1 -> swregin_4/2(data), swregin_3/2(data), swregin_2/2(data), swregin_1/2(data), swregin_/2(data)
  swregin_1/1(dataout) -> Out2/1
  addr/1 -> swregin_3/1(address), swregin_4/1(address), swregin_2/1(address), swregin_1/1(address), swregin_/1(address)
  swregin_/1(dataout) -> Out1/1
  Constant9/1 -> swregin_2/3(myaddress)
  swregin_3/1(dataout) -> Out4/1
  Constant8/1 -> swregin_1/3(myaddress)

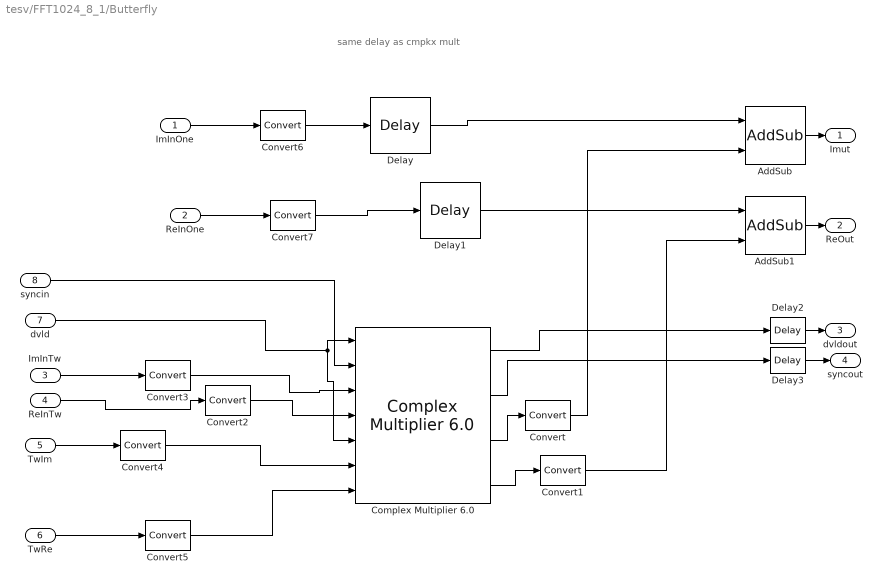
== system tesv/FFT1024_8_1/Butterfly ==
  note: same delay as cmpkx mult
  ImInOne : Inport
  ReInOne : Inport  Port=2
  ImInTw : Inport  Port=3
  ReInTw : Inport  Port=4
  TwIm : Inport  Port=5
  TwRe : Inport  Port=6
  dvld : Inport  Port=7
  syncin : Inport  Port=8
  AddSub : xbsIndex_r4/AddSub  mode=Addition  use_carryin=off  use_carryout=off  en=off  latency=1  precision=Full  arith_type=Unsigned  n_bits=16  bin_pt=14  quantization=Truncate  overflow=Wrap  use_behavioral_HDL=off  hw_selection=Fabric  pipelined=off  dbl_ovrd=off  block_type=addsub
  AddSub1 : xbsIndex_r4/AddSub  mode=Addition  use_carryin=off  use_carryout=off  en=off  latency=1  precision=Full  arith_type=Unsigned  n_bits=16  bin_pt=14  quantization=Truncate  overflow=Wrap  use_behavioral_HDL=off  hw_selection=Fabric  pipelined=off  dbl_ovrd=off  block_type=addsub
  "Complex Multiplier 6.0 " : xbsIndex_r4/Complex Multiplier 6.0   hasatlast=on  hasatuser=off  atuserwidth=1  hasbtlast=off  hasbtuser=off  btuserwidth=1  multtype=Use_Mults  optimizegoal=Resources  flowcontrol=NonBlocking  outputwidth=18  roundmode=Truncate  hasctrltlast=off  hasctrltuser=off  ctrltuserwidth=1  outtlastbehv=Pass_A_TLAST  latencyconfig=Automatic  minimumlatency=37  aclken=off  aresetn=off  trim_axipin_name=on  simulation_type=hybrid_sim  simulation_model=sysgen:cmpy_v6_0  data_path_portlist={ 's_axis_a_tdata_real', 's_axis_a_tdata_imag', 's_axis_b_tdata_real', 's_axis_b_tdata_imag', 's_axis_ctrl_tdata_rounding_bit', 'm_axis_dout_tdata_real', 'm_axis_dout_tdata_imag' }  aportwidth=63  bportwidth=63  ip_name=Complex Multiplier  ip_version=6.0  dsptool_ready=true  ipcore_usecache=true  ipcore_useipmodelcache=true  ipcore_verbose=false  ipcore_latency_parameter='minimumlatency'  wrapper_available=true  port_translation_map={ 'aclken' => 'en', 'aresetn' => 'rst'}  block_type=cmpy_v6_0
  Convert{,1..7} (8 alike) : xbsIndex_r4/Convert  gui_display_data_type=Fixed-point  arith_type="Signed  (2's comp)"  n_bits=16  bin_pt=14  float_type=Single  exp_bits=8  fraction_bits=24  quantization=Truncate  overflow=Wrap  en=off  latency=0  pipeline=off  dbl_ovrd=off  block_type=convert
  Delay : xbsIndex_r4/Delay  rst=off  infoeditControl=Selection of Reset will increase slice count due to use of real FFs and instead of SRLs  en=off  latency=6  reg_retiming=off  dbl_ovrd=off  block_type=delay
  Delay1 : xbsIndex_r4/Delay  rst=off  infoeditControl=Selection of Reset will increase slice count due to use of real FFs and instead of SRLs  en=off  latency=6  reg_retiming=off  dbl_ovrd=off  block_type=delay
  Delay2 : xbsIndex_r4/Delay  rst=off  infoeditControl=Selection of Reset will increase slice count due to use of real FFs and instead of SRLs  en=off  latency=1  reg_retiming=off  dbl_ovrd=off  block_type=delay
  Delay3 : xbsIndex_r4/Delay  rst=off  infoeditControl=Selection of Reset will increase slice count due to use of real FFs and instead of SRLs  en=off  latency=1  reg_retiming=off  dbl_ovrd=off  block_type=delay
  Imut : Outport
  ReOut : Outport  Port=2
  dvldout : Outport  Port=3
  syncout : Outport  Port=4
  wires:
  ReInOne/1 -> Convert7/1
  ImInOne/1 -> Convert6/1
  AddSub/1 -> Imut/1
  AddSub1/1 -> ReOut/1
  ImInTw/1 -> Convert3/1
  ReInTw/1 -> Convert2/1
  Delay/1 -> AddSub/1
  Delay1/1 -> AddSub1/1
  TwIm/1 -> Convert4/1
  TwRe/1 -> Convert5/1
  dvld/1 -> "Complex Multiplier 6.0 "/1, "Complex Multiplier 6.0 "/5
  Convert6/1 -> Delay/1
  Convert7/1 -> Delay1/1
  Convert3/1 -> "Complex Multiplier 6.0 "/3
  Convert2/1 -> "Complex Multiplier 6.0 "/4
  Convert4/1 -> "Complex Multiplier 6.0 "/6
  Convert5/1 -> "Complex Multiplier 6.0 "/7
  Convert1/1 -> AddSub1/2
  syncin/1 -> "Complex Multiplier 6.0 "/2
  "Complex Multiplier 6.0 "/4 -> Convert1/1
  "Complex Multiplier 6.0 "/3 -> Convert/1
  "Complex Multiplier 6.0 "/1 -> Delay2/1
  "Complex Multiplier 6.0 "/2 -> Delay3/1
  Convert/1 -> AddSub/2
  Delay2/1 -> dvldout/1
  Delay3/1 -> syncout/1

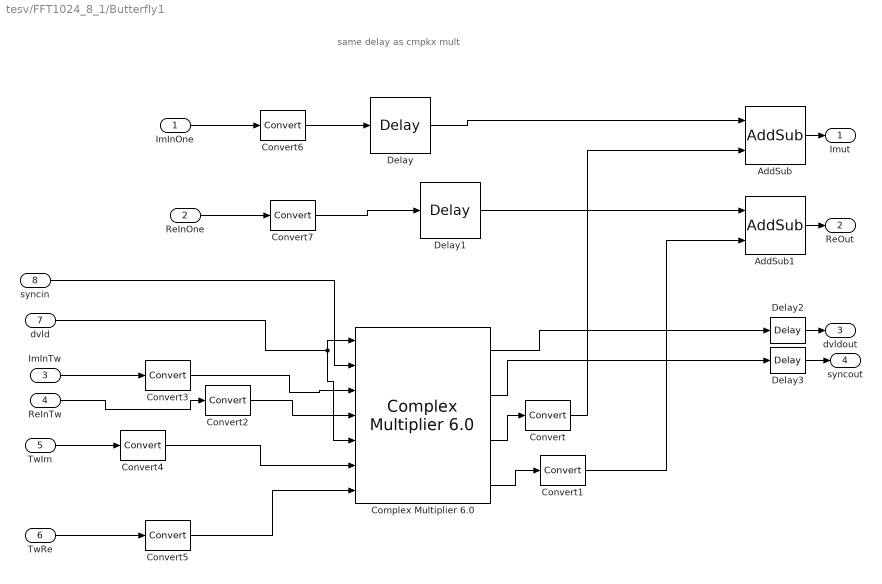
== system tesv/FFT1024_8_1/Butterfly1 ==
  note: same delay as cmpkx mult
  ImInOne : Inport
  ReInOne : Inport  Port=2
  ImInTw : Inport  Port=3
  ReInTw : Inport  Port=4
  TwIm : Inport  Port=5
  TwRe : Inport  Port=6
  dvld : Inport  Port=7
  syncin : Inport  Port=8
  AddSub : xbsIndex_r4/AddSub  mode=Addition  use_carryin=off  use_carryout=off  en=off  latency=1  precision=Full  arith_type=Unsigned  n_bits=16  bin_pt=14  quantization=Truncate  overflow=Wrap  use_behavioral_HDL=off  hw_selection=Fabric  pipelined=off  dbl_ovrd=off  block_type=addsub
  AddSub1 : xbsIndex_r4/AddSub  mode=Addition  use_carryin=off  use_carryout=off  en=off  latency=1  precision=Full  arith_type=Unsigned  n_bits=16  bin_pt=14  quantization=Truncate  overflow=Wrap  use_behavioral_HDL=off  hw_selection=Fabric  pipelined=off  dbl_ovrd=off  block_type=addsub
  "Complex Multiplier 6.0 " : xbsIndex_r4/Complex Multiplier 6.0   hasatlast=on  hasatuser=off  atuserwidth=1  hasbtlast=off  hasbtuser=off  btuserwidth=1  multtype=Use_Mults  optimizegoal=Resources  flowcontrol=NonBlocking  outputwidth=18  roundmode=Truncate  hasctrltlast=off  hasctrltuser=off  ctrltuserwidth=1  outtlastbehv=Pass_A_TLAST  latencyconfig=Automatic  minimumlatency=37  aclken=off  aresetn=off  trim_axipin_name=on  simulation_type=hybrid_sim  simulation_model=sysgen:cmpy_v6_0  data_path_portlist={ 's_axis_a_tdata_real', 's_axis_a_tdata_imag', 's_axis_b_tdata_real', 's_axis_b_tdata_imag', 's_axis_ctrl_tdata_rounding_bit', 'm_axis_dout_tdata_real', 'm_axis_dout_tdata_imag' }  aportwidth=63  bportwidth=63  ip_name=Complex Multiplier  ip_version=6.0  dsptool_ready=true  ipcore_usecache=true  ipcore_useipmodelcache=true  ipcore_verbose=false  ipcore_latency_parameter='minimumlatency'  wrapper_available=true  port_translation_map={ 'aclken' => 'en', 'aresetn' => 'rst'}  block_type=cmpy_v6_0
  Convert{,1..7} (8 alike) : xbsIndex_r4/Convert  gui_display_data_type=Fixed-point  arith_type="Signed  (2's comp)"  n_bits=16  bin_pt=14  float_type=Single  exp_bits=8  fraction_bits=24  quantization=Truncate  overflow=Wrap  en=off  latency=0  pipeline=off  dbl_ovrd=off  block_type=convert
  Delay : xbsIndex_r4/Delay  rst=off  infoeditControl=Selection of Reset will increase slice count due to use of real FFs and instead of SRLs  en=off  latency=6  reg_retiming=off  dbl_ovrd=off  block_type=delay
  Delay1 : xbsIndex_r4/Delay  rst=off  infoeditControl=Selection of Reset will increase slice count due to use of real FFs and instead of SRLs  en=off  latency=6  reg_retiming=off  dbl_ovrd=off  block_type=delay
  Delay2 : xbsIndex_r4/Delay  rst=off  infoeditControl=Selection of Reset will increase slice count due to use of real FFs and instead of SRLs  en=off  latency=1  reg_retiming=off  dbl_ovrd=off  block_type=delay
  Delay3 : xbsIndex_r4/Delay  rst=off  infoeditControl=Selection of Reset will increase slice count due to use of real FFs and instead of SRLs  en=off  latency=1  reg_retiming=off  dbl_ovrd=off  block_type=delay
  Imut : Outport
  ReOut : Outport  Port=2
  dvldout : Outport  Port=3
  syncout : Outport  Port=4
  wires:
  ReInOne/1 -> Convert7/1
  ImInOne/1 -> Convert6/1
  AddSub/1 -> Imut/1
  AddSub1/1 -> ReOut/1
  ImInTw/1 -> Convert3/1
  ReInTw/1 -> Convert2/1
  Delay/1 -> AddSub/1
  Delay1/1 -> AddSub1/1
  TwIm/1 -> Convert4/1
  TwRe/1 -> Convert5/1
  dvld/1 -> "Complex Multiplier 6.0 "/1, "Complex Multiplier 6.0 "/5
  Convert6/1 -> Delay/1
  Convert7/1 -> Delay1/1
  Convert3/1 -> "Complex Multiplier 6.0 "/3
  Convert2/1 -> "Complex Multiplier 6.0 "/4
  Convert4/1 -> "Complex Multiplier 6.0 "/6
  Convert5/1 -> "Complex Multiplier 6.0 "/7
  Convert1/1 -> AddSub1/2
  syncin/1 -> "Complex Multiplier 6.0 "/2
  "Complex Multiplier 6.0 "/4 -> Convert1/1
  "Complex Multiplier 6.0 "/3 -> Convert/1
  "Complex Multiplier 6.0 "/1 -> Delay2/1
  "Complex Multiplier 6.0 "/2 -> Delay3/1
  Convert/1 -> AddSub/2
  Delay2/1 -> dvldout/1
  Delay3/1 -> syncout/1

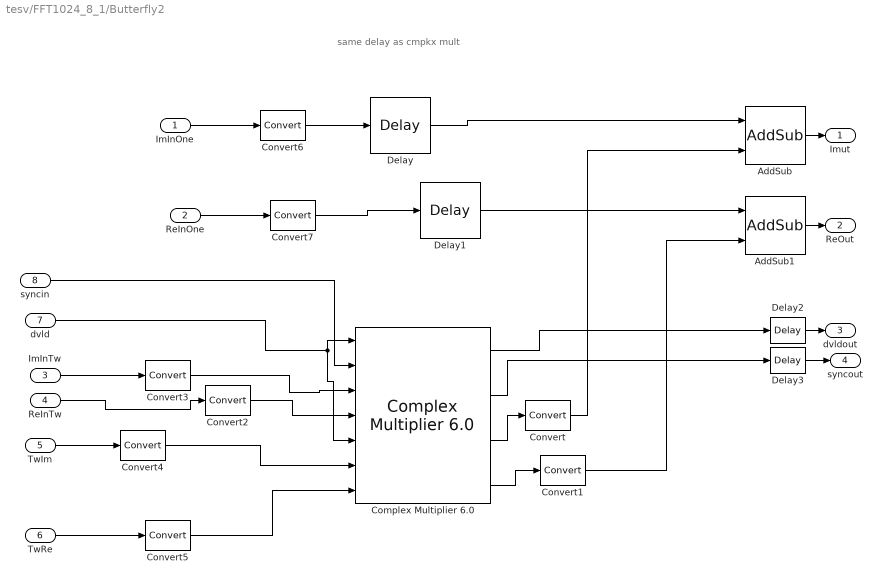
== system tesv/FFT1024_8_1/Butterfly2 ==
  note: same delay as cmpkx mult
  ImInOne : Inport
  ReInOne : Inport  Port=2
  ImInTw : Inport  Port=3
  ReInTw : Inport  Port=4
  TwIm : Inport  Port=5
  TwRe : Inport  Port=6
  dvld : Inport  Port=7
  syncin : Inport  Port=8
  AddSub : xbsIndex_r4/AddSub  mode=Addition  use_carryin=off  use_carryout=off  en=off  latency=1  precision=Full  arith_type=Unsigned  n_bits=16  bin_pt=14  quantization=Truncate  overflow=Wrap  use_behavioral_HDL=off  hw_selection=Fabric  pipelined=off  dbl_ovrd=off  block_type=addsub
  AddSub1 : xbsIndex_r4/AddSub  mode=Addition  use_carryin=off  use_carryout=off  en=off  latency=1  precision=Full  arith_type=Unsigned  n_bits=16  bin_pt=14  quantization=Truncate  overflow=Wrap  use_behavioral_HDL=off  hw_selection=Fabric  pipelined=off  dbl_ovrd=off  block_type=addsub
  "Complex Multiplier 6.0 " : xbsIndex_r4/Complex Multiplier 6.0   hasatlast=on  hasatuser=off  atuserwidth=1  hasbtlast=off  hasbtuser=off  btuserwidth=1  multtype=Use_Mults  optimizegoal=Resources  flowcontrol=NonBlocking  outputwidth=18  roundmode=Truncate  hasctrltlast=off  hasctrltuser=off  ctrltuserwidth=1  outtlastbehv=Pass_A_TLAST  latencyconfig=Automatic  minimumlatency=37  aclken=off  aresetn=off  trim_axipin_name=on  simulation_type=hybrid_sim  simulation_model=sysgen:cmpy_v6_0  data_path_portlist={ 's_axis_a_tdata_real', 's_axis_a_tdata_imag', 's_axis_b_tdata_real', 's_axis_b_tdata_imag', 's_axis_ctrl_tdata_rounding_bit', 'm_axis_dout_tdata_real', 'm_axis_dout_tdata_imag' }  aportwidth=63  bportwidth=63  ip_name=Complex Multiplier  ip_version=6.0  dsptool_ready=true  ipcore_usecache=true  ipcore_useipmodelcache=true  ipcore_verbose=false  ipcore_latency_parameter='minimumlatency'  wrapper_available=true  port_translation_map={ 'aclken' => 'en', 'aresetn' => 'rst'}  block_type=cmpy_v6_0
  Convert{,1..7} (8 alike) : xbsIndex_r4/Convert  gui_display_data_type=Fixed-point  arith_type="Signed  (2's comp)"  n_bits=16  bin_pt=14  float_type=Single  exp_bits=8  fraction_bits=24  quantization=Truncate  overflow=Wrap  en=off  latency=0  pipeline=off  dbl_ovrd=off  block_type=convert
  Delay : xbsIndex_r4/Delay  rst=off  infoeditControl=Selection of Reset will increase slice count due to use of real FFs and instead of SRLs  en=off  latency=6  reg_retiming=off  dbl_ovrd=off  block_type=delay
  Delay1 : xbsIndex_r4/Delay  rst=off  infoeditControl=Selection of Reset will increase slice count due to use of real FFs and instead of SRLs  en=off  latency=6  reg_retiming=off  dbl_ovrd=off  block_type=delay
  Delay2 : xbsIndex_r4/Delay  rst=off  infoeditControl=Selection of Reset will increase slice count due to use of real FFs and instead of SRLs  en=off  latency=1  reg_retiming=off  dbl_ovrd=off  block_type=delay
  Delay3 : xbsIndex_r4/Delay  rst=off  infoeditControl=Selection of Reset will increase slice count due to use of real FFs and instead of SRLs  en=off  latency=1  reg_retiming=off  dbl_ovrd=off  block_type=delay
  Imut : Outport
  ReOut : Outport  Port=2
  dvldout : Outport  Port=3
  syncout : Outport  Port=4
  wires:
  ReInOne/1 -> Convert7/1
  ImInOne/1 -> Convert6/1
  AddSub/1 -> Imut/1
  AddSub1/1 -> ReOut/1
  ImInTw/1 -> Convert3/1
  ReInTw/1 -> Convert2/1
  Delay/1 -> AddSub/1
  Delay1/1 -> AddSub1/1
  TwIm/1 -> Convert4/1
  TwRe/1 -> Convert5/1
  dvld/1 -> "Complex Multiplier 6.0 "/1, "Complex Multiplier 6.0 "/5
  Convert6/1 -> Delay/1
  Convert7/1 -> Delay1/1
  Convert3/1 -> "Complex Multiplier 6.0 "/3
  Convert2/1 -> "Complex Multiplier 6.0 "/4
  Convert4/1 -> "Complex Multiplier 6.0 "/6
  Convert5/1 -> "Complex Multiplier 6.0 "/7
  Convert1/1 -> AddSub1/2
  syncin/1 -> "Complex Multiplier 6.0 "/2
  "Complex Multiplier 6.0 "/4 -> Convert1/1
  "Complex Multiplier 6.0 "/3 -> Convert/1
  "Complex Multiplier 6.0 "/1 -> Delay2/1
  "Complex Multiplier 6.0 "/2 -> Delay3/1
  Convert/1 -> AddSub/2
  Delay2/1 -> dvldout/1
  Delay3/1 -> syncout/1
